simulink model "model_demo"  (R2023b)
settings: Solver=VariableStepAuto  StartTime=0.0  StopTime=10.0  RelTol=1e-3
undefined symbols (not defined in the file): DiscIntNeverNeededParam, magnitude, Newton, Raphson
libraries: simulink x61, slpidlib x19
(part 3 of 3)

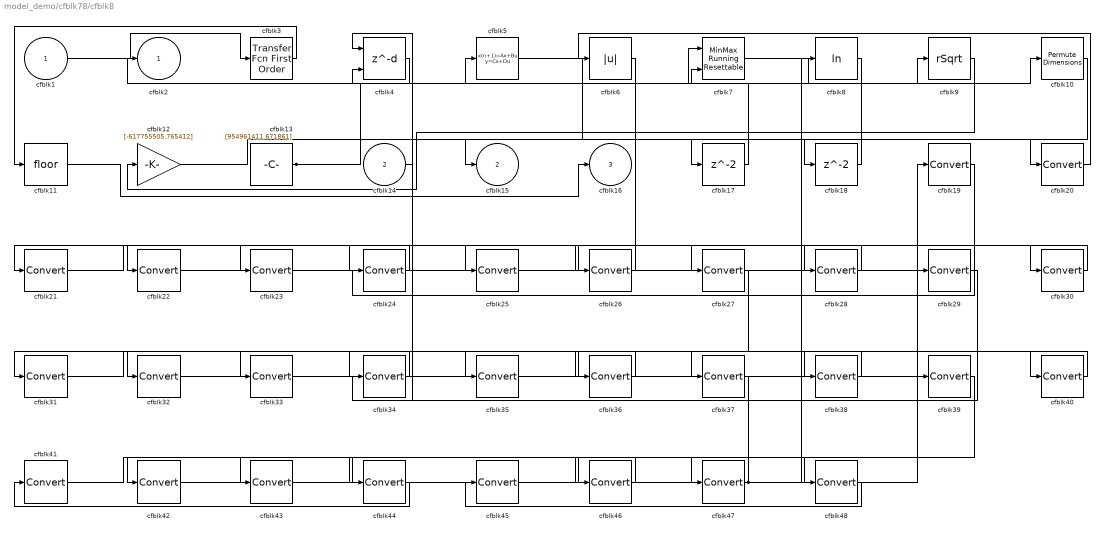
== system model_demo/cfblk78/cfblk8 ==
  cfblk1 : Inport
  cfblk14 : Inport  Port=2
  cfblk10 : PermuteDimensions
  cfblk11 : Rounding
  cfblk12 : Gain  Gain=[-617755505.765412]
  cfblk13 : Constant  Value=[954961411.671861]  SampleTime=1
  cfblk17 : Delay  SampleTime=1
  cfblk18 : Delay  SampleTime=1
  cfblk{19..48} (30 alike) : DataTypeConversion  SaturateOnIntegerOverflow=off  RndMeth=Floor
  cfblk3 : simulink/Discrete/Transfer Fcn First Order  PoleZ=0.95  ICPrevOutput=0.0  DoSatur=off
  cfblk4 : Delay  DelayLengthSource=Input port  SampleTime=1
      settings: InputPortMap=u0,p1
  cfblk5 : DiscreteStateSpace
  cfblk6 : Abs  SaturateOnIntegerOverflow=off
  cfblk7 : simulink/Math Operations/MinMax Running Resettable  Function=min  vinit=0.0
  cfblk8 : Math  Operator=log
  cfblk9 : Sqrt  Operator=rSqrt  AlgorithmType=Newton-Raphson
  cfblk2 : Outport
  cfblk15 : Outport  Port=2
  cfblk16 : Outport  Port=3
  wires:
  cfblk10/1 -> cfblk15/1
  cfblk1/1 -> cfblk3/1
  cfblk4/1 -> cfblk2/1
  cfblk14/1 -> cfblk4/1
  cfblk3/1 -> cfblk11/1
  cfblk7/1 -> cfblk9/1
  cfblk9/1 -> cfblk12/1
  cfblk13/1 -> cfblk10/1, cfblk7/2
  cfblk11/1 -> cfblk16/1
  cfblk8/1 -> cfblk17/1
  cfblk17/1 -> cfblk5/1
  cfblk12/1 -> cfblk18/1
  cfblk18/1 -> cfblk7/1
  cfblk5/1 -> cfblk20/1
  cfblk20/1 -> cfblk6/1
  cfblk6/1 -> cfblk22/1
  cfblk22/1 -> cfblk19/1
  cfblk19/1 -> cfblk24/1
  cfblk24/1 -> cfblk21/1
  cfblk21/1 -> cfblk26/1
  cfblk26/1 -> cfblk23/1
  cfblk23/1 -> cfblk28/1
  cfblk28/1 -> cfblk25/1
  cfblk25/1 -> cfblk30/1
  cfblk30/1 -> cfblk27/1
  cfblk27/1 -> cfblk32/1
  cfblk32/1 -> cfblk29/1
  cfblk29/1 -> cfblk34/1
  cfblk34/1 -> cfblk31/1
  cfblk31/1 -> cfblk36/1
  cfblk36/1 -> cfblk33/1
  cfblk33/1 -> cfblk38/1
  cfblk38/1 -> cfblk35/1
  cfblk35/1 -> cfblk40/1
  cfblk40/1 -> cfblk37/1
  cfblk37/1 -> cfblk42/1
  cfblk42/1 -> cfblk39/1
  cfblk39/1 -> cfblk44/1
  cfblk44/1 -> cfblk41/1
  cfblk45/1 -> cfblk47/1
  cfblk41/1 -> cfblk46/1
  cfblk46/1 -> cfblk43/1
  cfblk47/1 -> cfblk8/1, cfblk4/2
  cfblk43/1 -> cfblk48/1
  cfblk48/1 -> cfblk45/1

== system model_demo/cfblk79/cfblk12 ==
  cfblk1 : Inport
  cfblk3 : simulink/Discrete/Transfer Fcn Real Zero  ZeroZ=0.75  ICPrevInput=0.0  DoSatur=off
  cfblk4 : ComplexToMagnitudeAngle
  cfblk5 : ComplexToMagnitudeAngle
  cfblk6 : Sum  Inputs=--
  cfblk8 : Delay  SampleTime=1
  cfblk2 : Outport
  cfblk7 : Outport  Port=2
  wires:
  cfblk5/1 -> cfblk7/1
  cfblk3/1 -> cfblk4/1
  cfblk5/2 -> cfblk6/1
  cfblk1/1 -> cfblk2/1
  cfblk4/1 -> cfblk5/1
  cfblk4/2 -> cfblk6/2
  cfblk6/1 -> cfblk8/1
  cfblk8/1 -> cfblk3/1

== system model_demo/cfblk80/cfblk6 ==
  cfblk1 : Inport
  cfblk10 : Constant  Value=[956331216.469066]  SampleTime=1
  cfblk12 : Delay  SampleTime=1
  cfblk3 : Delay  DelayLengthSource=Input port  SampleTime=1
      settings: InputPortMap=u0,p1
  cfblk4 : Sum  Inputs=+
  cfblk5 : Sum  Inputs=+
  cfblk6 : Abs  SaturateOnIntegerOverflow=off
  cfblk7 : Sum  Inputs=|++
  cfblk8 : Sqrt
  cfblk9 : Assignment  DiagnosticForDimensions=Warning  IndexOptions=Index vector (dialog)  Indices=1  OutputSizes=1
  cfblk2 : Outport
  cfblk11 : Outport  Port=2
  wires:
  cfblk10/1 -> cfblk8/1, cfblk9/1
  cfblk1/1 -> cfblk3/1
  cfblk5/1 -> cfblk3/2
  cfblk3/1 -> cfblk2/1, cfblk11/1
  cfblk4/1 -> cfblk7/1, cfblk9/2
  cfblk6/1 -> cfblk5/1
  cfblk9/1 -> cfblk7/2
  cfblk8/1 -> cfblk6/1
  cfblk7/1 -> cfblk12/1
  cfblk12/1 -> cfblk4/1

== system model_demo/cfblk80/cfblk7 ==
  cfblk1 : Inport
  cfblk9 : Inport  Port=2
  cfblk10 : Delay  SampleTime=1
  cfblk3 : simulink/Discrete/Transfer Fcn Real Zero  ZeroZ=0.75  ICPrevInput=0.0  DoSatur=off
  cfblk4 : DiscreteZeroPole  Poles=[0 0.5]  Gain=1
  cfblk5 : Delay  SampleTime=1
  cfblk6 : Sum  Inputs=+
  cfblk7 : Sum  Inputs=+
  cfblk8 : Constant  Value=[-3888514.740939]  SampleTime=1
  cfblk2 : Outport
  wires:
  cfblk6/1 -> cfblk2/1
  cfblk1/1 -> cfblk5/1
  cfblk3/1 -> cfblk4/1
  cfblk8/1 -> cfblk6/1
  cfblk4/1 -> cfblk7/1
  cfblk7/1 -> cfblk10/1
  cfblk10/1 -> cfblk3/1

== system model_demo/cfblk80/cfblk8 ==
  cfblk1 : Inport
  cfblk9 : Inport  Port=2
  cfblk10 : Inport  Port=3
  cfblk3 : slpidlib/PID Controller (2DOF)  Controller=PID  Form=Parallel  TimeDomain=Discrete-time  UseExternalTs=off  SampleTime=1  IntegratorMethod=Forward Euler  FilterMethod=Forward Euler  ControllerParametersSource=internal  P=1  I=1  UseKiTs=off  D=0  N=100  UseFilter=on  b=1  c=1  TunerSelectOption=Transfer Function Based (PID Tuner App)  InitialConditionSource=internal  InitialConditionForIntegrator=0  InitialConditionForFilter=0  DifferentiatorICPrevScaledInput=0  ExternalReset=none  TrackingMode=off  Kt=1  LimitOutput=off  SatLimitsSource=internal  UpperSaturationLimit=inf  LowerSaturationLimit=-inf  LinearizeAsGain=off  AntiWindupMode=none  Kb=1  LimitIntegrator=off  UpperIntegratorSaturationLimit=inf  LowerIntegratorSaturationLimit=-inf  POutMin=[]  POutMax=[]  IOutMin=[]  IOutMax=[]  DOutMin=[]  DOutMax=[]  NOutMin=[]  NOutMax=[]  bOutMin=[]  bOutMax=[]  cOutMin=[]  cOutMax=[]  SumOutMin=[]  SumOutMax=[]  SaturationOutMin=[]  SaturationOutMax=[]  PParamMin=[]  PParamMax=[]  IParamMin=[]  IParamMax=[]  DParamMin=[]  DParamMax=[]  NParamMin=[]  NParamMax=[]  bParamMin=[]  bParamMax=[]  cParamMin=[]  cParamMax=[]  KbParamMin=[]  KbParamMax=[]  KtParamMin=[]  KtParamMax=[]  KbOutMin=[]  KbOutMax=[]  KtOutMin=[]  KtOutMax=[]  IntegratorOutMin=[]  IntegratorOutMax=[]  FilterOutMin=[]  FilterOutMax=[]  SumI1OutMin=[]  SumI1OutMax=[]  SumI2OutMin=[]  SumI2OutMax=[]  SumI3OutMin=[]  SumI3OutMax=[]  SumI4OutMin=[]  SumI4OutMax=[]  SumDOutMin=[]  SumDOutMax=[]  Sum1OutMin=[]  Sum1OutMax=[]  Sum2OutMin=[]  Sum2OutMax=[]  Sum3OutMin=[]  Sum3OutMax=[]  DifferentiatorOutMin=[]  DifferentiatorOutMax=[]  FilterDiffOutCoefMin=[]  FilterDiffOutCoefMax=[]  ReciprocalOutMin=[]  ReciprocalOutMax=[]  SumDenOutMin=[]  SumDenOutMax=[]  SumNumOutMin=[]  SumNumOutMax=[]  DivideOutMin=[]  DivideOutMax=[]  UdiffTsProdOutMin=[]  UdiffTsProdOutMax=[]  NTsProdOutMin=[]  NTsProdOutMax=[]  UintegralTsProdOutMin=[]  UintegralTsProdOutMax=[]  UngainTsProdOutMin=[]  UngainTsProdOutMax=[]  ClampingZeroOutDataTypeStr=Inherit: Inherit via back propagation  ClampingZeroOutMin=[]  ClampingZeroOutMax=[]  FilterDenConstantOutDataTypeStr=Inherit: Inherit via back propagation  FilterDenConstantOutMin=[]  FilterDenConstantOutMax=[]  PCopyOutDataTypeStr=Inherit: Inherit via back propagation  PCopyOutMin=[]  PCopyOutMax=[]  NCopyOutDataTypeStr=Inherit: Inherit via back propagation  NCopyOutMin=[]  NCopyOutMax=[]  IntegratorContinuousStateAttributes=''  IntegratorStateMustResolveToSignalObject=off  IntegratorRTWStateStorageClass=Auto  FilterContinuousStateAttributes=''  FilterStateMustResolveToSignalObject=off  FilterRTWStateStorageClass=Auto  ParallelPVariant=InternalParameters  IdealPVariant=Disabled  IVariant=InternalParameters  DVariant=InternalParameters  bVariant=InternalParameters  cVariant=InternalParameters  IntegratorVariant=Discrete  SatVariant=Disabled  AWVariant=Passthrough  PCopyVariant=Disabled  TRVariant=Disabled  FdbkBlocksVariant=Forward  IdealPFdbkVariant=Disabled  SatFdbkVariant=Disabled  DerivativeFilterVariant=ForwardEulerFilter  NVariant=InternalParameters  NCopyVariant=Disabled  FilterICVariant=InternalICsFilter  IntegratorICVariant=InternalICs  ExternalResetVariant=Disabled  TRSumVariant=Passthrough  SumFdbkVariant=Disabled  SumVariant=Sum_PID  TsampFilterVariant=InternalTs  TsampNgainVariant=Passthrough  TsampIntegralVariant=Disabled_SignalSpec  ExternalSaturationOutDataTypeStr=Inherit: Same as second input
      settings: LibrarySourceBlock=simulink/Discrete/Discrete PID Controller (2DOF)
  cfblk4 : Delay  DelayLengthSource=Input port  SampleTime=1
      settings: InputPortMap=u0,p1
  cfblk5 : Sum  Inputs=+
  cfblk6 : MinMax  Function=max  Inputs=3
  cfblk7 : Product  Inputs=*
  cfblk8 : Constant  Value=[999994514.434890]  SampleTime=1
  cfblk2 : Outport
  cfblk11 : Outport  Port=2
  cfblk12 : Outport  Port=3
  wires:
  cfblk6/1 -> cfblk11/1
  cfblk3/1 -> cfblk6/1, cfblk4/2
  cfblk10/1 -> cfblk3/1
  cfblk4/1 -> cfblk12/1
  cfblk7/1 -> cfblk3/2
  cfblk1/1 -> cfblk6/2
  cfblk9/1 -> cfblk4/1, cfblk5/1
  cfblk5/1 -> cfblk6/3, cfblk2/1
  cfblk8/1 -> cfblk7/1

== system model_demo/cfblk80/cfblk9 ==
  cfblk1 : Inport
  cfblk12 : Inport  Port=2
  cfblk13 : Inport  Port=3
  cfblk10 : Constant  Value=[680607672.793325]  SampleTime=1
  cfblk11 : Constant  Value=[263129341.713534]  SampleTime=1
  cfblk3 : PropagationDelay  SampleTime=1
  cfblk4 : UnaryMinus
  cfblk5 : Sqrt
  cfblk6 : Signum
  cfblk7 : PermuteDimensions
  cfblk8 : Trigonometry
  cfblk9 : Constant  Value=[217539892.668750]  SampleTime=1
  cfblk2 : Outport
  wires:
  cfblk7/1 -> cfblk4/1
  cfblk3/1 -> cfblk2/1
  cfblk13/1 -> cfblk5/1
  cfblk4/1 -> cfblk8/1
  cfblk11/1 -> cfblk7/1
  cfblk1/1 -> cfblk3/1
  cfblk12/1 -> cfblk6/1
  cfblk6/1 -> cfblk3/2

== system model_demo/cfblk81/cfblk10 ==
  cfblk1 : Inport
  cfblk6 : Inport  Port=2
  cfblk3 : MinMax  Inputs=3
  cfblk4 : Sum  Inputs=-+
  cfblk5 : Sqrt  Operator=rSqrt  AlgorithmType=Newton-Raphson
  cfblk2 : Outport
  cfblk7 : Outport  Port=2
  wires:
  cfblk4/1 -> cfblk2/1
  cfblk1/1 -> cfblk7/1, cfblk3/3
  cfblk6/1 -> cfblk5/1, cfblk4/2
  cfblk5/1 -> cfblk3/1, cfblk3/2
  cfblk3/1 -> cfblk4/1

== system model_demo/cfblk81/cfblk11 ==
  cfblk1 : Inport
  cfblk8 : Inport  Port=2
  cfblk9 : Inport  Port=3
  cfblk10 : Inport  Port=4
  cfblk3 : simulink/Discrete/Transfer Fcn Lead or Lag  PoleZ=0.95  ZeroZ=0.75  ICPrevOutput=0.0  ICPrevInput=0.0  DoSatur=off
  cfblk4 : Assignment  DiagnosticForDimensions=Warning  IndexOptions=Index vector (dialog)  Indices=1  OutputSizes=1
  cfblk5 : ComplexToRealImag
  cfblk6 : Bias  Bias=[8664871.233920]  SaturateOnIntegerOverflow=off
  cfblk7 : Rounding
  cfblk2 : Outport
  cfblk11 : Outport  Port=2
  wires:
  cfblk6/1 -> cfblk3/1
  cfblk5/1 -> cfblk11/1
  cfblk9/1 -> cfblk2/1
  cfblk10/1 -> cfblk7/1
  cfblk5/2 -> cfblk6/1
  cfblk8/1 -> cfblk4/1
  cfblk1/1 -> cfblk5/1
  cfblk3/1 -> cfblk4/2

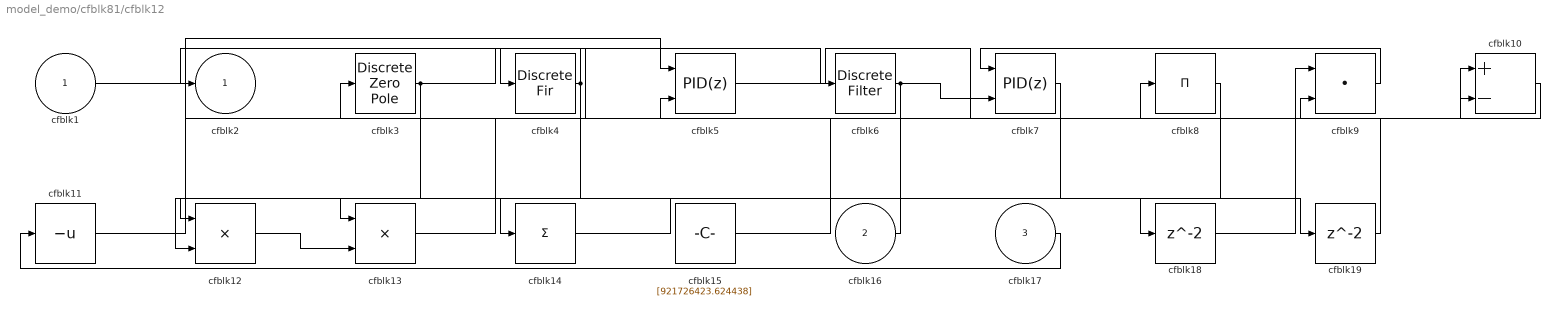
== system model_demo/cfblk81/cfblk12 ==
  cfblk1 : Inport
  cfblk16 : Inport  Port=2
  cfblk17 : Inport  Port=3
  cfblk10 : Sum  Inputs=+-
  cfblk11 : UnaryMinus
  cfblk12 : Product
  cfblk13 : Product
  cfblk14 : Sum  Inputs=+
  cfblk15 : Constant  Value=[921726423.624438]  SampleTime=1
  cfblk18 : Delay  SampleTime=1
  cfblk19 : Delay  SampleTime=1
  cfblk3 : DiscreteZeroPole  Poles=[0 0.5]  Gain=1
  cfblk4 : DiscreteFir  SampleTime=1
  cfblk5 : slpidlib/PID Controller (2DOF)  Controller=PID  Form=Parallel  TimeDomain=Discrete-time  UseExternalTs=off  SampleTime=1  IntegratorMethod=Forward Euler  FilterMethod=Forward Euler  ControllerParametersSource=internal  P=1  I=1  UseKiTs=off  D=0  N=100  UseFilter=on  b=1  c=1  TunerSelectOption=Transfer Function Based (PID Tuner App)  InitialConditionSource=internal  InitialConditionForIntegrator=0  InitialConditionForFilter=0  DifferentiatorICPrevScaledInput=0  ExternalReset=none  TrackingMode=off  Kt=1  LimitOutput=off  SatLimitsSource=internal  UpperSaturationLimit=inf  LowerSaturationLimit=-inf  LinearizeAsGain=off  AntiWindupMode=none  Kb=1  LimitIntegrator=off  UpperIntegratorSaturationLimit=inf  LowerIntegratorSaturationLimit=-inf  POutMin=[]  POutMax=[]  IOutMin=[]  IOutMax=[]  DOutMin=[]  DOutMax=[]  NOutMin=[]  NOutMax=[]  bOutMin=[]  bOutMax=[]  cOutMin=[]  cOutMax=[]  SumOutMin=[]  SumOutMax=[]  SaturationOutMin=[]  SaturationOutMax=[]  PParamMin=[]  PParamMax=[]  IParamMin=[]  IParamMax=[]  DParamMin=[]  DParamMax=[]  NParamMin=[]  NParamMax=[]  bParamMin=[]  bParamMax=[]  cParamMin=[]  cParamMax=[]  KbParamMin=[]  KbParamMax=[]  KtParamMin=[]  KtParamMax=[]  KbOutMin=[]  KbOutMax=[]  KtOutMin=[]  KtOutMax=[]  IntegratorOutMin=[]  IntegratorOutMax=[]  FilterOutMin=[]  FilterOutMax=[]  SumI1OutMin=[]  SumI1OutMax=[]  SumI2OutMin=[]  SumI2OutMax=[]  SumI3OutMin=[]  SumI3OutMax=[]  SumI4OutMin=[]  SumI4OutMax=[]  SumDOutMin=[]  SumDOutMax=[]  Sum1OutMin=[]  Sum1OutMax=[]  Sum2OutMin=[]  Sum2OutMax=[]  Sum3OutMin=[]  Sum3OutMax=[]  DifferentiatorOutMin=[]  DifferentiatorOutMax=[]  FilterDiffOutCoefMin=[]  FilterDiffOutCoefMax=[]  ReciprocalOutMin=[]  ReciprocalOutMax=[]  SumDenOutMin=[]  SumDenOutMax=[]  SumNumOutMin=[]  SumNumOutMax=[]  DivideOutMin=[]  DivideOutMax=[]  UdiffTsProdOutMin=[]  UdiffTsProdOutMax=[]  NTsProdOutMin=[]  NTsProdOutMax=[]  UintegralTsProdOutMin=[]  UintegralTsProdOutMax=[]  UngainTsProdOutMin=[]  UngainTsProdOutMax=[]  ClampingZeroOutDataTypeStr=Inherit: Inherit via back propagation  ClampingZeroOutMin=[]  ClampingZeroOutMax=[]  FilterDenConstantOutDataTypeStr=Inherit: Inherit via back propagation  FilterDenConstantOutMin=[]  FilterDenConstantOutMax=[]  PCopyOutDataTypeStr=Inherit: Inherit via back propagation  PCopyOutMin=[]  PCopyOutMax=[]  NCopyOutDataTypeStr=Inherit: Inherit via back propagation  NCopyOutMin=[]  NCopyOutMax=[]  IntegratorContinuousStateAttributes=''  IntegratorStateMustResolveToSignalObject=off  IntegratorRTWStateStorageClass=Auto  FilterContinuousStateAttributes=''  FilterStateMustResolveToSignalObject=off  FilterRTWStateStorageClass=Auto  ParallelPVariant=InternalParameters  IdealPVariant=Disabled  IVariant=InternalParameters  DVariant=InternalParameters  bVariant=InternalParameters  cVariant=InternalParameters  IntegratorVariant=Discrete  SatVariant=Disabled  AWVariant=Passthrough  PCopyVariant=Disabled  TRVariant=Disabled  FdbkBlocksVariant=Forward  IdealPFdbkVariant=Disabled  SatFdbkVariant=Disabled  DerivativeFilterVariant=ForwardEulerFilter  NVariant=InternalParameters  NCopyVariant=Disabled  FilterICVariant=InternalICsFilter  IntegratorICVariant=InternalICs  ExternalResetVariant=Disabled  TRSumVariant=Passthrough  SumFdbkVariant=Disabled  SumVariant=Sum_PID  TsampFilterVariant=InternalTs  TsampNgainVariant=Passthrough  TsampIntegralVariant=Disabled_SignalSpec  ExternalSaturationOutDataTypeStr=Inherit: Same as second input
      settings: LibrarySourceBlock=simulink/Discrete/Discrete PID Controller (2DOF)
  cfblk6 : DiscreteFilter  SampleTime=1
  cfblk7 : slpidlib/PID Controller (2DOF)  Controller=PID  Form=Parallel  TimeDomain=Discrete-time  UseExternalTs=off  SampleTime=1  IntegratorMethod=Forward Euler  FilterMethod=Forward Euler  ControllerParametersSource=internal  P=1  I=1  UseKiTs=off  D=0  N=100  UseFilter=on  b=1  c=1  TunerSelectOption=Transfer Function Based (PID Tuner App)  InitialConditionSource=internal  InitialConditionForIntegrator=0  InitialConditionForFilter=0  DifferentiatorICPrevScaledInput=0  ExternalReset=none  TrackingMode=off  Kt=1  LimitOutput=off  SatLimitsSource=internal  UpperSaturationLimit=inf  LowerSaturationLimit=-inf  LinearizeAsGain=off  AntiWindupMode=none  Kb=1  LimitIntegrator=off  UpperIntegratorSaturationLimit=inf  LowerIntegratorSaturationLimit=-inf  POutMin=[]  POutMax=[]  IOutMin=[]  IOutMax=[]  DOutMin=[]  DOutMax=[]  NOutMin=[]  NOutMax=[]  bOutMin=[]  bOutMax=[]  cOutMin=[]  cOutMax=[]  SumOutMin=[]  SumOutMax=[]  SaturationOutMin=[]  SaturationOutMax=[]  PParamMin=[]  PParamMax=[]  IParamMin=[]  IParamMax=[]  DParamMin=[]  DParamMax=[]  NParamMin=[]  NParamMax=[]  bParamMin=[]  bParamMax=[]  cParamMin=[]  cParamMax=[]  KbParamMin=[]  KbParamMax=[]  KtParamMin=[]  KtParamMax=[]  KbOutMin=[]  KbOutMax=[]  KtOutMin=[]  KtOutMax=[]  IntegratorOutMin=[]  IntegratorOutMax=[]  FilterOutMin=[]  FilterOutMax=[]  SumI1OutMin=[]  SumI1OutMax=[]  SumI2OutMin=[]  SumI2OutMax=[]  SumI3OutMin=[]  SumI3OutMax=[]  SumI4OutMin=[]  SumI4OutMax=[]  SumDOutMin=[]  SumDOutMax=[]  Sum1OutMin=[]  Sum1OutMax=[]  Sum2OutMin=[]  Sum2OutMax=[]  Sum3OutMin=[]  Sum3OutMax=[]  DifferentiatorOutMin=[]  DifferentiatorOutMax=[]  FilterDiffOutCoefMin=[]  FilterDiffOutCoefMax=[]  ReciprocalOutMin=[]  ReciprocalOutMax=[]  SumDenOutMin=[]  SumDenOutMax=[]  SumNumOutMin=[]  SumNumOutMax=[]  DivideOutMin=[]  DivideOutMax=[]  UdiffTsProdOutMin=[]  UdiffTsProdOutMax=[]  NTsProdOutMin=[]  NTsProdOutMax=[]  UintegralTsProdOutMin=[]  UintegralTsProdOutMax=[]  UngainTsProdOutMin=[]  UngainTsProdOutMax=[]  ClampingZeroOutDataTypeStr=Inherit: Inherit via back propagation  ClampingZeroOutMin=[]  ClampingZeroOutMax=[]  FilterDenConstantOutDataTypeStr=Inherit: Inherit via back propagation  FilterDenConstantOutMin=[]  FilterDenConstantOutMax=[]  PCopyOutDataTypeStr=Inherit: Inherit via back propagation  PCopyOutMin=[]  PCopyOutMax=[]  NCopyOutDataTypeStr=Inherit: Inherit via back propagation  NCopyOutMin=[]  NCopyOutMax=[]  IntegratorContinuousStateAttributes=''  IntegratorStateMustResolveToSignalObject=off  IntegratorRTWStateStorageClass=Auto  FilterContinuousStateAttributes=''  FilterStateMustResolveToSignalObject=off  FilterRTWStateStorageClass=Auto  ParallelPVariant=InternalParameters  IdealPVariant=Disabled  IVariant=InternalParameters  DVariant=InternalParameters  bVariant=InternalParameters  cVariant=InternalParameters  IntegratorVariant=Discrete  SatVariant=Disabled  AWVariant=Passthrough  PCopyVariant=Disabled  TRVariant=Disabled  FdbkBlocksVariant=Forward  IdealPFdbkVariant=Disabled  SatFdbkVariant=Disabled  DerivativeFilterVariant=ForwardEulerFilter  NVariant=InternalParameters  NCopyVariant=Disabled  FilterICVariant=InternalICsFilter  IntegratorICVariant=InternalICs  ExternalResetVariant=Disabled  TRSumVariant=Passthrough  SumFdbkVariant=Disabled  SumVariant=Sum_PID  TsampFilterVariant=InternalTs  TsampNgainVariant=Passthrough  TsampIntegralVariant=Disabled_SignalSpec  ExternalSaturationOutDataTypeStr=Inherit: Same as second input
      settings: LibrarySourceBlock=simulink/Discrete/Discrete PID Controller (2DOF)
  cfblk8 : Product  Inputs=*
  cfblk9 : DotProduct  OutDataTypeStr=Inherit: Inherit via internal rule
  cfblk2 : Outport
  wires:
  cfblk9/1 -> cfblk7/1
  cfblk16/1 -> cfblk4/1
  cfblk5/1 -> cfblk8/1
  cfblk11/1 -> cfblk5/1
  cfblk10/1 -> cfblk5/2
  cfblk3/1 -> cfblk13/1, cfblk6/1
  cfblk1/1 -> cfblk9/2
  cfblk6/1 -> cfblk14/1, cfblk7/2
  cfblk4/1 -> cfblk12/1, cfblk2/1
  cfblk12/1 -> cfblk13/2
  cfblk15/1 -> cfblk10/1
  cfblk13/1 -> cfblk10/2
  cfblk7/1 -> cfblk12/2
  cfblk17/1 -> cfblk11/1
  cfblk8/1 -> cfblk18/1
  cfblk18/1 -> cfblk9/1
  cfblk14/1 -> cfblk19/1
  cfblk19/1 -> cfblk3/1

== system model_demo/cfblk81/cfblk13 ==
  cfblk1 : Inport
  cfblk10 : Inport  Port=2
  cfblk11 : Inport  Port=3
  cfblk14 : Delay  SampleTime=1
  cfblk3 : simulink/Discrete/Transfer Fcn First Order  PoleZ=0.95  ICPrevOutput=0.0  DoSatur=off
  cfblk4 : simulink/Discrete/Transfer Fcn First Order  PoleZ=0.95  ICPrevOutput=0.0  DoSatur=off
  cfblk5 : DiscreteTransferFcn  SampleTime=1
  cfblk6 : simulink/Discrete/Transfer Fcn Real Zero  ZeroZ=0.75  ICPrevInput=0.0  DoSatur=off
  cfblk7 : UnaryMinus
  cfblk8 : Reshape
  cfblk9 : Squeeze
  cfblk2 : Outport
  cfblk12 : Outport  Port=2
  cfblk13 : Outport  Port=3
  wires:
  cfblk4/1 -> cfblk2/1
  cfblk5/1 -> cfblk9/1
  cfblk10/1 -> cfblk12/1
  cfblk6/1 -> cfblk7/1
  cfblk7/1 -> cfblk13/1
  cfblk3/1 -> cfblk6/1
  cfblk11/1 -> cfblk4/1
  cfblk1/1 -> cfblk8/1
  cfblk8/1 -> cfblk3/1
  cfblk9/1 -> cfblk14/1
  cfblk14/1 -> cfblk5/1

== system model_demo/cfblk81/cfblk14 ==
  cfblk1 : Inport
  cfblk14 : Inport  Port=2
  cfblk10 : Polyval  Coefs=[ +2.081618890e-019, -1.441693666e-014, +4.719686976e-010, -8.536869453e-006, +1.621573104e-001, -8.087801117e+001 ]
  cfblk11 : Product  Inputs=**
  cfblk12 : PermuteDimensions
  cfblk13 : Constant  Value=[-781974819.007084]  SampleTime=1
  cfblk3 : slpidlib/PID Controller (2DOF)  Controller=PID  Form=Parallel  TimeDomain=Discrete-time  UseExternalTs=off  SampleTime=1  IntegratorMethod=Forward Euler  FilterMethod=Forward Euler  ControllerParametersSource=internal  P=1  I=1  UseKiTs=off  D=0  N=100  UseFilter=on  b=1  c=1  TunerSelectOption=Transfer Function Based (PID Tuner App)  InitialConditionSource=internal  InitialConditionForIntegrator=0  InitialConditionForFilter=0  DifferentiatorICPrevScaledInput=0  ExternalReset=none  TrackingMode=off  Kt=1  LimitOutput=off  SatLimitsSource=internal  UpperSaturationLimit=inf  LowerSaturationLimit=-inf  LinearizeAsGain=off  AntiWindupMode=none  Kb=1  LimitIntegrator=off  UpperIntegratorSaturationLimit=inf  LowerIntegratorSaturationLimit=-inf  POutMin=[]  POutMax=[]  IOutMin=[]  IOutMax=[]  DOutMin=[]  DOutMax=[]  NOutMin=[]  NOutMax=[]  bOutMin=[]  bOutMax=[]  cOutMin=[]  cOutMax=[]  SumOutMin=[]  SumOutMax=[]  SaturationOutMin=[]  SaturationOutMax=[]  PParamMin=[]  PParamMax=[]  IParamMin=[]  IParamMax=[]  DParamMin=[]  DParamMax=[]  NParamMin=[]  NParamMax=[]  bParamMin=[]  bParamMax=[]  cParamMin=[]  cParamMax=[]  KbParamMin=[]  KbParamMax=[]  KtParamMin=[]  KtParamMax=[]  KbOutMin=[]  KbOutMax=[]  KtOutMin=[]  KtOutMax=[]  IntegratorOutMin=[]  IntegratorOutMax=[]  FilterOutMin=[]  FilterOutMax=[]  SumI1OutMin=[]  SumI1OutMax=[]  SumI2OutMin=[]  SumI2OutMax=[]  SumI3OutMin=[]  SumI3OutMax=[]  SumI4OutMin=[]  SumI4OutMax=[]  SumDOutMin=[]  SumDOutMax=[]  Sum1OutMin=[]  Sum1OutMax=[]  Sum2OutMin=[]  Sum2OutMax=[]  Sum3OutMin=[]  Sum3OutMax=[]  DifferentiatorOutMin=[]  DifferentiatorOutMax=[]  FilterDiffOutCoefMin=[]  FilterDiffOutCoefMax=[]  ReciprocalOutMin=[]  ReciprocalOutMax=[]  SumDenOutMin=[]  SumDenOutMax=[]  SumNumOutMin=[]  SumNumOutMax=[]  DivideOutMin=[]  DivideOutMax=[]  UdiffTsProdOutMin=[]  UdiffTsProdOutMax=[]  NTsProdOutMin=[]  NTsProdOutMax=[]  UintegralTsProdOutMin=[]  UintegralTsProdOutMax=[]  UngainTsProdOutMin=[]  UngainTsProdOutMax=[]  ClampingZeroOutDataTypeStr=Inherit: Inherit via back propagation  ClampingZeroOutMin=[]  ClampingZeroOutMax=[]  FilterDenConstantOutDataTypeStr=Inherit: Inherit via back propagation  FilterDenConstantOutMin=[]  FilterDenConstantOutMax=[]  PCopyOutDataTypeStr=Inherit: Inherit via back propagation  PCopyOutMin=[]  PCopyOutMax=[]  NCopyOutDataTypeStr=Inherit: Inherit via back propagation  NCopyOutMin=[]  NCopyOutMax=[]  IntegratorContinuousStateAttributes=''  IntegratorStateMustResolveToSignalObject=off  IntegratorRTWStateStorageClass=Auto  FilterContinuousStateAttributes=''  FilterStateMustResolveToSignalObject=off  FilterRTWStateStorageClass=Auto  ParallelPVariant=InternalParameters  IdealPVariant=Disabled  IVariant=InternalParameters  DVariant=InternalParameters  bVariant=InternalParameters  cVariant=InternalParameters  IntegratorVariant=Discrete  SatVariant=Disabled  AWVariant=Passthrough  PCopyVariant=Disabled  TRVariant=Disabled  FdbkBlocksVariant=Forward  IdealPFdbkVariant=Disabled  SatFdbkVariant=Disabled  DerivativeFilterVariant=ForwardEulerFilter  NVariant=InternalParameters  NCopyVariant=Disabled  FilterICVariant=InternalICsFilter  IntegratorICVariant=InternalICs  ExternalResetVariant=Disabled  TRSumVariant=Passthrough  SumFdbkVariant=Disabled  SumVariant=Sum_PID  TsampFilterVariant=InternalTs  TsampNgainVariant=Passthrough  TsampIntegralVariant=Disabled_SignalSpec  ExternalSaturationOutDataTypeStr=Inherit: Same as second input
      settings: LibrarySourceBlock=simulink/Discrete/Discrete PID Controller (2DOF)
  cfblk4 : simulink/Discrete/Transfer Fcn Real Zero  ZeroZ=0.75  ICPrevInput=0.0  DoSatur=off
  cfblk5 : DiscreteZeroPole  Poles=[0 0.5]  Gain=1
  cfblk6 : DiscreteStateSpace
  cfblk7 : Abs  SaturateOnIntegerOverflow=off
  cfblk8 : Trigonometry
  cfblk9 : Math  Operator=log10
  cfblk2 : Outport
  cfblk15 : Outport  Port=2
  cfblk16 : Outport  Port=3
  wires:
  cfblk13/1 -> cfblk11/1, cfblk12/1
  cfblk8/1 -> cfblk4/1
  cfblk3/1 -> cfblk6/1
  cfblk12/1 -> cfblk10/1
  cfblk7/1 -> cfblk2/1
  cfblk5/1 -> cfblk16/1, cfblk3/2
  cfblk6/1 -> cfblk15/1
  cfblk9/1 -> cfblk7/1
  cfblk1/1 -> cfblk11/2
  cfblk14/1 -> cfblk5/1
  cfblk10/1 -> cfblk9/1
  cfblk11/1 -> cfblk8/1
  cfblk4/1 -> cfblk3/1

== system model_demo/cfblk81/cfblk9 ==
  cfblk1 : Inport
  cfblk7 : Inport  Port=2
  cfblk8 : Inport  Port=3
  cfblk10 : Delay  SampleTime=1
  cfblk3 : simulink/Discrete/Transfer Fcn Lead or Lag  PoleZ=0.95  ZeroZ=0.75  ICPrevOutput=0.0  ICPrevInput=0.0  DoSatur=off
  cfblk4 : Sin  TimeSource=Use external signal  SampleTime=0
  cfblk5 : Abs  SaturateOnIntegerOverflow=off
  cfblk6 : MinMax  Function=max  Inputs=3
  cfblk2 : Outport
  cfblk9 : Outport  Port=2
  wires:
  cfblk7/1 -> cfblk2/1
  cfblk3/1 -> cfblk4/1
  cfblk5/1 -> cfblk9/1, cfblk10/1
  cfblk8/1 -> cfblk6/1
  cfblk6/1 -> cfblk5/1
  cfblk4/1 -> cfblk6/2
  cfblk1/1 -> cfblk3/1
  cfblk10/1 -> cfblk6/3

== system model_demo/cfblk82/cfblk12 ==
  cfblk1 : Inport
  cfblk11 : Inport  Port=2
  cfblk12 : Inport  Port=3
  cfblk13 : Inport  Port=4
  cfblk14 : Inport  Port=5
  cfblk15 : Inport  Port=6
  cfblk10 : Constant  Value=[345707446.991535]  SampleTime=1
  cfblk3 : Delay  ShowEnablePort=on  SampleTime=1
      settings: InputPortMap=u0,e6
  cfblk4 : simulink/Discrete/Transfer Fcn First Order  PoleZ=0.95  ICPrevOutput=0.0  DoSatur=off
  cfblk5 : slpidlib/PID Controller (2DOF)  Controller=PID  Form=Parallel  TimeDomain=Discrete-time  UseExternalTs=off  SampleTime=1  IntegratorMethod=Forward Euler  FilterMethod=Forward Euler  ControllerParametersSource=internal  P=1  I=1  UseKiTs=off  D=0  N=100  UseFilter=on  b=1  c=1  TunerSelectOption=Transfer Function Based (PID Tuner App)  InitialConditionSource=internal  InitialConditionForIntegrator=0  InitialConditionForFilter=0  DifferentiatorICPrevScaledInput=0  ExternalReset=none  TrackingMode=off  Kt=1  LimitOutput=off  SatLimitsSource=internal  UpperSaturationLimit=inf  LowerSaturationLimit=-inf  LinearizeAsGain=off  AntiWindupMode=none  Kb=1  LimitIntegrator=off  UpperIntegratorSaturationLimit=inf  LowerIntegratorSaturationLimit=-inf  POutMin=[]  POutMax=[]  IOutMin=[]  IOutMax=[]  DOutMin=[]  DOutMax=[]  NOutMin=[]  NOutMax=[]  bOutMin=[]  bOutMax=[]  cOutMin=[]  cOutMax=[]  SumOutMin=[]  SumOutMax=[]  SaturationOutMin=[]  SaturationOutMax=[]  PParamMin=[]  PParamMax=[]  IParamMin=[]  IParamMax=[]  DParamMin=[]  DParamMax=[]  NParamMin=[]  NParamMax=[]  bParamMin=[]  bParamMax=[]  cParamMin=[]  cParamMax=[]  KbParamMin=[]  KbParamMax=[]  KtParamMin=[]  KtParamMax=[]  KbOutMin=[]  KbOutMax=[]  KtOutMin=[]  KtOutMax=[]  IntegratorOutMin=[]  IntegratorOutMax=[]  FilterOutMin=[]  FilterOutMax=[]  SumI1OutMin=[]  SumI1OutMax=[]  SumI2OutMin=[]  SumI2OutMax=[]  SumI3OutMin=[]  SumI3OutMax=[]  SumI4OutMin=[]  SumI4OutMax=[]  SumDOutMin=[]  SumDOutMax=[]  Sum1OutMin=[]  Sum1OutMax=[]  Sum2OutMin=[]  Sum2OutMax=[]  Sum3OutMin=[]  Sum3OutMax=[]  DifferentiatorOutMin=[]  DifferentiatorOutMax=[]  FilterDiffOutCoefMin=[]  FilterDiffOutCoefMax=[]  ReciprocalOutMin=[]  ReciprocalOutMax=[]  SumDenOutMin=[]  SumDenOutMax=[]  SumNumOutMin=[]  SumNumOutMax=[]  DivideOutMin=[]  DivideOutMax=[]  UdiffTsProdOutMin=[]  UdiffTsProdOutMax=[]  NTsProdOutMin=[]  NTsProdOutMax=[]  UintegralTsProdOutMin=[]  UintegralTsProdOutMax=[]  UngainTsProdOutMin=[]  UngainTsProdOutMax=[]  ClampingZeroOutDataTypeStr=Inherit: Inherit via back propagation  ClampingZeroOutMin=[]  ClampingZeroOutMax=[]  FilterDenConstantOutDataTypeStr=Inherit: Inherit via back propagation  FilterDenConstantOutMin=[]  FilterDenConstantOutMax=[]  PCopyOutDataTypeStr=Inherit: Inherit via back propagation  PCopyOutMin=[]  PCopyOutMax=[]  NCopyOutDataTypeStr=Inherit: Inherit via back propagation  NCopyOutMin=[]  NCopyOutMax=[]  IntegratorContinuousStateAttributes=''  IntegratorStateMustResolveToSignalObject=off  IntegratorRTWStateStorageClass=Auto  FilterContinuousStateAttributes=''  FilterStateMustResolveToSignalObject=off  FilterRTWStateStorageClass=Auto  ParallelPVariant=InternalParameters  IdealPVariant=Disabled  IVariant=InternalParameters  DVariant=InternalParameters  bVariant=InternalParameters  cVariant=InternalParameters  IntegratorVariant=Discrete  SatVariant=Disabled  AWVariant=Passthrough  PCopyVariant=Disabled  TRVariant=Disabled  FdbkBlocksVariant=Forward  IdealPFdbkVariant=Disabled  SatFdbkVariant=Disabled  DerivativeFilterVariant=ForwardEulerFilter  NVariant=InternalParameters  NCopyVariant=Disabled  FilterICVariant=InternalICsFilter  IntegratorICVariant=InternalICs  ExternalResetVariant=Disabled  TRSumVariant=Passthrough  SumFdbkVariant=Disabled  SumVariant=Sum_PID  TsampFilterVariant=InternalTs  TsampNgainVariant=Passthrough  TsampIntegralVariant=Disabled_SignalSpec  ExternalSaturationOutDataTypeStr=Inherit: Same as second input
      settings: LibrarySourceBlock=simulink/Discrete/Discrete PID Controller (2DOF)
  cfblk6 : Sum  Inputs=+-
  cfblk7 : Product  Inputs=**
  cfblk8 : Product
  cfblk9 : Constant  Value=[806755621.526693]  SampleTime=1
  cfblk2 : Outport
  cfblk16 : Outport  Port=2
  wires:
  cfblk9/1 -> cfblk8/1
  cfblk14/1 -> cfblk6/1
  cfblk1/1 -> cfblk4/1
  cfblk4/1 -> cfblk16/1
  cfblk5/1 -> cfblk2/1
  cfblk7/1 -> cfblk6/2
  cfblk12/1 -> cfblk8/2
  cfblk11/1 -> cfblk7/1
  cfblk6/1 -> cfblk3/1
  cfblk13/1 -> cfblk7/2
  cfblk3/1 -> cfblk5/1
  cfblk15/1 -> cfblk5/2
  cfblk8/1 -> cfblk3/2

== system model_demo/cfblk82/cfblk13 ==
  cfblk1 : Inport
  cfblk6 : Inport  Port=2
  cfblk3 : simulink/Discrete/Transfer Fcn First Order  PoleZ=0.95  ICPrevOutput=0.0  DoSatur=off
  cfblk4 : simulink/Discrete/Transfer Fcn Lead or Lag  PoleZ=0.95  ZeroZ=0.75  ICPrevOutput=0.0  ICPrevInput=0.0  DoSatur=off
  cfblk5 : simulink/Math Operations/Slider Gain  gain=1  low=0  high=2
  cfblk2 : Outport
  cfblk7 : Outport  Port=2
  wires:
  cfblk4/1 -> cfblk5/1
  cfblk5/1 -> cfblk2/1
  cfblk6/1 -> cfblk3/1
  cfblk1/1 -> cfblk7/1
  cfblk3/1 -> cfblk4/1

== system model_demo/cfblk82/cfblk14 ==
  cfblk1 : Inport
  cfblk7 : Inport  Port=2
  cfblk8 : Inport  Port=3
  cfblk9 : Inport  Port=4
  cfblk10 : Delay  SampleTime=1
  cfblk3 : Delay  DelayLengthSource=Input port  SampleTime=1
      settings: InputPortMap=u0,p1
  cfblk4 : Delay  DelayLengthSource=Input port  SampleTime=1
      settings: InputPortMap=u0,p1
  cfblk5 : Polyval  Coefs=[ +2.081618890e-019, -1.441693666e-014, +4.719686976e-010, -8.536869453e-006, +1.621573104e-001, -8.087801117e+001 ]
  cfblk6 : Gain  Gain=[424032298.343210]
  cfblk2 : Outport
  wires:
  cfblk8/1 -> cfblk2/1
  cfblk5/1 -> cfblk4/1
  cfblk1/1 -> cfblk4/2
  cfblk7/1 -> cfblk5/1
  cfblk3/1 -> cfblk6/1
  cfblk9/1 -> cfblk3/2
  cfblk6/1 -> cfblk10/1
  cfblk10/1 -> cfblk3/1

== system model_demo/cfblk82/cfblk18 ==
  cfblk1 : Inport
  cfblk7 : Inport  Port=2
  cfblk8 : Inport  Port=3
  Action Port : ActionPort  ActionPortLabel=if(u1 >= 0)
  cfblk3 : simulink/Discrete/Difference  ICPrevInput=0.0  OutMin=[]  OutMax=[]  OutDataTypeStr=Inherit: Inherit via back propagation  OutDataType=fixdt(1, 16)  OutScaling=2^-10  DoSatur=off
  cfblk4 : slpidlib/PID Controller (2DOF)  Controller=PID  Form=Parallel  TimeDomain=Discrete-time  UseExternalTs=off  SampleTime=-1  IntegratorMethod=Forward Euler  FilterMethod=Forward Euler  ControllerParametersSource=internal  P=1  I=1  UseKiTs=off  D=0  N=100  UseFilter=on  b=1  c=1  TunerSelectOption=Transfer Function Based (PID Tuner App)  InitialConditionSource=internal  InitialConditionForIntegrator=0  InitialConditionForFilter=0  DifferentiatorICPrevScaledInput=0  ExternalReset=none  TrackingMode=off  Kt=1  LimitOutput=off  SatLimitsSource=internal  UpperSaturationLimit=inf  LowerSaturationLimit=-inf  LinearizeAsGain=off  AntiWindupMode=none  Kb=1  LimitIntegrator=off  UpperIntegratorSaturationLimit=inf  LowerIntegratorSaturationLimit=-inf  POutMin=[]  POutMax=[]  IOutMin=[]  IOutMax=[]  DOutMin=[]  DOutMax=[]  NOutMin=[]  NOutMax=[]  bOutMin=[]  bOutMax=[]  cOutMin=[]  cOutMax=[]  SumOutMin=[]  SumOutMax=[]  SaturationOutMin=[]  SaturationOutMax=[]  PParamMin=[]  PParamMax=[]  IParamMin=[]  IParamMax=[]  DParamMin=[]  DParamMax=[]  NParamMin=[]  NParamMax=[]  bParamMin=[]  bParamMax=[]  cParamMin=[]  cParamMax=[]  KbParamMin=[]  KbParamMax=[]  KtParamMin=[]  KtParamMax=[]  KbOutMin=[]  KbOutMax=[]  KtOutMin=[]  KtOutMax=[]  IntegratorOutMin=[]  IntegratorOutMax=[]  FilterOutMin=[]  FilterOutMax=[]  SumI1OutMin=[]  SumI1OutMax=[]  SumI2OutMin=[]  SumI2OutMax=[]  SumI3OutMin=[]  SumI3OutMax=[]  SumI4OutMin=[]  SumI4OutMax=[]  SumDOutMin=[]  SumDOutMax=[]  Sum1OutMin=[]  Sum1OutMax=[]  Sum2OutMin=[]  Sum2OutMax=[]  Sum3OutMin=[]  Sum3OutMax=[]  DifferentiatorOutMin=[]  DifferentiatorOutMax=[]  FilterDiffOutCoefMin=[]  FilterDiffOutCoefMax=[]  ReciprocalOutMin=[]  ReciprocalOutMax=[]  SumDenOutMin=[]  SumDenOutMax=[]  SumNumOutMin=[]  SumNumOutMax=[]  DivideOutMin=[]  DivideOutMax=[]  UdiffTsProdOutMin=[]  UdiffTsProdOutMax=[]  NTsProdOutMin=[]  NTsProdOutMax=[]  UintegralTsProdOutMin=[]  UintegralTsProdOutMax=[]  UngainTsProdOutMin=[]  UngainTsProdOutMax=[]  ClampingZeroOutDataTypeStr=Inherit: Inherit via back propagation  ClampingZeroOutMin=[]  ClampingZeroOutMax=[]  FilterDenConstantOutDataTypeStr=Inherit: Inherit via back propagation  FilterDenConstantOutMin=[]  FilterDenConstantOutMax=[]  PCopyOutDataTypeStr=Inherit: Inherit via back propagation  PCopyOutMin=[]  PCopyOutMax=[]  NCopyOutDataTypeStr=Inherit: Inherit via back propagation  NCopyOutMin=[]  NCopyOutMax=[]  IntegratorContinuousStateAttributes=''  IntegratorStateMustResolveToSignalObject=off  IntegratorRTWStateStorageClass=Auto  FilterContinuousStateAttributes=''  FilterStateMustResolveToSignalObject=off  FilterRTWStateStorageClass=Auto  ParallelPVariant=InternalParameters  IdealPVariant=Disabled  IVariant=InternalParameters  DVariant=InternalParameters  bVariant=InternalParameters  cVariant=InternalParameters  IntegratorVariant=Discrete  SatVariant=Disabled  AWVariant=Passthrough  PCopyVariant=Disabled  TRVariant=Disabled  FdbkBlocksVariant=Forward  IdealPFdbkVariant=Disabled  SatFdbkVariant=Disabled  DerivativeFilterVariant=ForwardEulerFilter  NVariant=InternalParameters  NCopyVariant=Disabled  FilterICVariant=InternalICsFilter  IntegratorICVariant=InternalICs  ExternalResetVariant=Disabled  TRSumVariant=Passthrough  SumFdbkVariant=Disabled  SumVariant=Sum_PID  TsampFilterVariant=InternalTs  TsampNgainVariant=Passthrough  TsampIntegralVariant=Disabled_SignalSpec  ExternalSaturationOutDataTypeStr=Inherit: Same as second input
      settings: LibrarySourceBlock=simulink/Discrete/Discrete PID Controller (2DOF)
  cfblk5 : Squeeze
  cfblk6 : Sum  Inputs=--
  cfblk2 : Outport
  wires:
  cfblk3/1 -> cfblk4/1
  cfblk1/1 -> cfblk2/1
  cfblk8/1 -> cfblk6/1
  cfblk5/1 -> cfblk6/2
  cfblk7/1 -> cfblk5/1, cfblk4/2
  cfblk6/1 -> cfblk3/1

== system model_demo/cfblk82/cfblk19 ==
  cfblk1 : Inport
  cfblk5 : Inport  Port=2
  cfblk6 : Inport  Port=3
  Action Port : ActionPort  ActionPortLabel=else
  cfblk3 : Delay
  cfblk4 : slpidlib/PID Controller  Controller=PID  Form=Parallel  TimeDomain=Discrete-time  UseExternalTs=off  SampleTime=-1  IntegratorMethod=Forward Euler  FilterMethod=Forward Euler  ControllerParametersSource=internal  P=1  I=1  UseKiTs=off  D=0  N=100  UseFilter=on  TunerSelectOption=Transfer Function Based (PID Tuner App)  InitialConditionSource=internal  InitialConditionForIntegrator=0  InitialConditionForFilter=0  DifferentiatorICPrevScaledInput=0  ExternalReset=none  TrackingMode=off  Kt=1  LimitOutput=off  SatLimitsSource=internal  UpperSaturationLimit=inf  LowerSaturationLimit=-inf  LinearizeAsGain=off  AntiWindupMode=none  Kb=1  LimitIntegrator=off  UpperIntegratorSaturationLimit=inf  LowerIntegratorSaturationLimit=-inf  POutMin=[]  POutMax=[]  IOutMin=[]  IOutMax=[]  DOutMin=[]  DOutMax=[]  NOutMin=[]  NOutMax=[]  SumOutMin=[]  SumOutMax=[]  SaturationOutMin=[]  SaturationOutMax=[]  PParamMin=[]  PParamMax=[]  IParamMin=[]  IParamMax=[]  DParamMin=[]  DParamMax=[]  NParamMin=[]  NParamMax=[]  KbParamMin=[]  KbParamMax=[]  KtParamMin=[]  KtParamMax=[]  KbOutMin=[]  KbOutMax=[]  KtOutMin=[]  KtOutMax=[]  IntegratorOutMin=[]  IntegratorOutMax=[]  FilterOutMin=[]  FilterOutMax=[]  SumI1OutMin=[]  SumI1OutMax=[]  SumI2OutMin=[]  SumI2OutMax=[]  SumI3OutMin=[]  SumI3OutMax=[]  SumI4OutMin=[]  SumI4OutMax=[]  SumDOutMin=[]  SumDOutMax=[]  DifferentiatorOutMin=[]  DifferentiatorOutMax=[]  FilterDiffOutCoefMin=[]  FilterDiffOutCoefMax=[]  ReciprocalOutMin=[]  ReciprocalOutMax=[]  SumDenOutMin=[]  SumDenOutMax=[]  SumNumOutMin=[]  SumNumOutMax=[]  DivideOutMin=[]  DivideOutMax=[]  UdiffTsProdOutMin=[]  UdiffTsProdOutMax=[]  NTsProdOutMin=[]  NTsProdOutMax=[]  UintegralTsProdOutMin=[]  UintegralTsProdOutMax=[]  UngainTsProdOutMin=[]  UngainTsProdOutMax=[]  ClampingZeroOutDataTypeStr=Inherit: Inherit via back propagation  ClampingZeroOutMin=[]  ClampingZeroOutMax=[]  FilterDenConstantOutDataTypeStr=Inherit: Inherit via back propagation  FilterDenConstantOutMin=[]  FilterDenConstantOutMax=[]  PCopyOutDataTypeStr=Inherit: Inherit via back propagation  PCopyOutMin=[]  PCopyOutMax=[]  NCopyOutDataTypeStr=Inherit: Inherit via back propagation  NCopyOutMin=[]  NCopyOutMax=[]  IntegratorContinuousStateAttributes=''  IntegratorStateMustResolveToSignalObject=off  IntegratorRTWStateStorageClass=Auto  FilterContinuousStateAttributes=''  FilterStateMustResolveToSignalObject=off  FilterRTWStateStorageClass=Auto  ParallelPVariant=InternalParameters  IdealPVariant=Disabled  IVariant=InternalParameters  DVariant=InternalParameters  IntegratorVariant=Discrete  SatVariant=Disabled  AWVariant=Passthrough  PCopyVariant=Disabled  TRVariant=Disabled  FdbkBlocksVariant=Forward  IdealPFdbkVariant=Disabled  SatFdbkVariant=Disabled  DerivativeFilterVariant=ForwardEulerFilter  NVariant=InternalParameters  NCopyVariant=Disabled  FilterICVariant=InternalICsFilter  IntegratorICVariant=InternalICs  ExternalResetVariant=Disabled  TRSumVariant=Passthrough  SumFdbkVariant=Disabled  SumVariant=Sum_PID  TsampFilterVariant=InternalTs  TsampNgainVariant=Passthrough  TsampIntegralVariant=Disabled_SignalSpec  ExternalSaturationOutDataTypeStr=Inherit: Same as second input
      settings: LibrarySourceBlock=simulink/Discrete/Discrete PID Controller
  cfblk2 : Outport
  cfblk7 : Outport  Port=2
  wires:
  cfblk6/1 -> cfblk3/1
  cfblk5/1 -> cfblk7/1
  cfblk4/1 -> cfblk2/1
  cfblk3/1 -> cfblk4/1

== system model_demo/cfblk83/cfblk7 ==
  cfblk1 : Inport
  cfblk9 : Inport  Port=2
  cfblk10 : Inport  Port=3
  cfblk11 : Inport  Port=4
  cfblk12 : Inport  Port=5
  cfblk3 : simulink/Discrete/Transfer Fcn Lead or Lag  PoleZ=0.95  ZeroZ=0.75  ICPrevOutput=0.0  ICPrevInput=0.0  DoSatur=off
  cfblk4 : simulink/Discrete/Difference  ICPrevInput=0.0  OutMin=[]  OutMax=[]  OutDataTypeStr=Inherit: Inherit via back propagation  OutDataType=fixdt(1, 16)  OutScaling=2^-10  DoSatur=off
  cfblk5 : DotProduct  OutDataTypeStr=Inherit: Inherit via internal rule
  cfblk6 : Signum
  cfblk7 : Constant  Value=[-754686844.111725]  SampleTime=1
  cfblk8 : Constant  Value=[225282182.475113]  SampleTime=1
  cfblk2 : Outport
  wires:
  cfblk10/1 -> cfblk6/1
  cfblk5/1 -> cfblk4/1
  cfblk1/1 -> cfblk5/1
  cfblk8/1 -> cfblk2/1
  cfblk4/1 -> cfblk3/1
  cfblk12/1 -> cfblk5/2

== system model_demo/cfblk83/cfblk8 ==
  cfblk1 : Inport
  cfblk8 : Inport  Port=2
  cfblk3 : Delay  DelayLengthSource=Input port  SampleTime=1
      settings: InputPortMap=u0,p1
  cfblk4 : DiscreteStateSpace
  cfblk5 : PropagationDelay  SampleTime=1
  cfblk6 : Abs  SaturateOnIntegerOverflow=off
  cfblk7 : Reshape
  cfblk9 : Delay  SampleTime=1
  cfblk2 : Outport
  wires:
  cfblk1/1 -> cfblk2/1
  cfblk4/1 -> cfblk7/1
  cfblk8/1 -> cfblk4/1
  cfblk3/1 -> cfblk5/1
  cfblk5/1 -> cfblk6/1
  cfblk7/1 -> cfblk3/1, cfblk3/2
  cfblk6/1 -> cfblk9/1
  cfblk9/1 -> cfblk5/2

== system model_demo/cfblk85/cfblk6 ==
  cfblk1 : Inport
  cfblk10 : Inport  Port=2
  cfblk11 : Inport  Port=3
  cfblk12 : Inport  Port=4
  cfblk14 : Delay
  cfblk3 : UnitDelay  SampleTime=-1  HasFrameUpgradeWarning=on
  cfblk4 : Polyval  Coefs=[ +2.081618890e-019, -1.441693666e-014, +4.719686976e-010, -8.536869453e-006, +1.621573104e-001, -8.087801117e+001 ]
  cfblk5 : Sqrt
  cfblk6 : PermuteDimensions
  cfblk7 : Sum  Inputs=+-
  cfblk8 : Sum  Inputs=|++
  cfblk9 : Constant  Value=[970697430.648301]  SampleTime=1
  cfblk2 : Outport
  cfblk13 : Outport  Port=2
  wires:
  cfblk9/1 -> cfblk13/1
  cfblk8/1 -> cfblk7/1
  cfblk4/1 -> cfblk6/1
  cfblk10/1 -> cfblk2/1
  cfblk12/1 -> cfblk7/2
  cfblk7/1 -> cfblk4/1
  cfblk11/1 -> cfblk8/1
  cfblk5/1 -> cfblk8/2
  cfblk3/1 -> cfblk5/1
  cfblk6/1 -> cfblk14/1
  cfblk14/1 -> cfblk3/1

== system model_demo/cfblk85/cfblk7 ==
  cfblk1 : Inport
  cfblk5 : Inport  Port=2
  cfblk6 : Inport  Port=3
  cfblk3 : UnaryMinus
  cfblk4 : Sum  Inputs=+-
  cfblk2 : Outport
  cfblk7 : Outport  Port=2
  wires:
  cfblk5/1 -> cfblk3/1
  cfblk6/1 -> cfblk4/1
  cfblk1/1 -> cfblk4/2
  cfblk4/1 -> cfblk2/1
  cfblk3/1 -> cfblk7/1

== system model_demo/cfblk85/cfblk8 ==
  cfblk1 : Inport
  cfblk10 : Inport  Port=2
  cfblk13 : Delay
  cfblk14 : Delay
  cfblk3 : DiscreteIntegrator  SampleTime=-1  ICPrevOutput=DiscIntNeverNeededParam  ICPrevScaledInput=DiscIntNeverNeededParam
  cfblk4 : Delay  DelayLengthSource=Input port
      settings: InputPortMap=u0,p1
  cfblk5 : DiscreteIntegrator  SampleTime=-1  ICPrevOutput=DiscIntNeverNeededParam  ICPrevScaledInput=DiscIntNeverNeededParam
  cfblk6 : Product
  cfblk7 : Signum
  cfblk8 : Rounding
  cfblk9 : Constant  Value=[715463942.614666]  SampleTime=1
  cfblk2 : Outport
  cfblk11 : Outport  Port=2
  cfblk12 : Outport  Port=3
  wires:
  cfblk3/1 -> cfblk7/1
  cfblk10/1 -> cfblk11/1
  cfblk7/1 -> cfblk8/1
  cfblk1/1 -> cfblk4/2
  cfblk4/1 -> cfblk3/1
  cfblk5/1 -> cfblk12/1, cfblk6/2
  cfblk9/1 -> cfblk2/1, cfblk6/1
  cfblk8/1 -> cfblk13/1
  cfblk13/1 -> cfblk4/1
  cfblk6/1 -> cfblk14/1
  cfblk14/1 -> cfblk5/1

== system model_demo/cfblk86/cfblk6 ==
  cfblk1 : Inport
  cfblk8 : Inport  Port=2
  cfblk9 : Inport  Port=3
  cfblk10 : Inport  Port=4
  cfblk11 : Inport  Port=5
  cfblk12 : Inport  Port=6
  cfblk3 : slpidlib/PID Controller  Controller=PID  Form=Parallel  TimeDomain=Discrete-time  UseExternalTs=off  SampleTime=-1  IntegratorMethod=Forward Euler  FilterMethod=Forward Euler  ControllerParametersSource=internal  P=1  I=1  UseKiTs=off  D=0  N=100  UseFilter=on  TunerSelectOption=Transfer Function Based (PID Tuner App)  InitialConditionSource=internal  InitialConditionForIntegrator=0  InitialConditionForFilter=0  DifferentiatorICPrevScaledInput=0  ExternalReset=none  TrackingMode=off  Kt=1  LimitOutput=off  SatLimitsSource=internal  UpperSaturationLimit=inf  LowerSaturationLimit=-inf  LinearizeAsGain=off  AntiWindupMode=none  Kb=1  LimitIntegrator=off  UpperIntegratorSaturationLimit=inf  LowerIntegratorSaturationLimit=-inf  POutMin=[]  POutMax=[]  IOutMin=[]  IOutMax=[]  DOutMin=[]  DOutMax=[]  NOutMin=[]  NOutMax=[]  SumOutMin=[]  SumOutMax=[]  SaturationOutMin=[]  SaturationOutMax=[]  PParamMin=[]  PParamMax=[]  IParamMin=[]  IParamMax=[]  DParamMin=[]  DParamMax=[]  NParamMin=[]  NParamMax=[]  KbParamMin=[]  KbParamMax=[]  KtParamMin=[]  KtParamMax=[]  KbOutMin=[]  KbOutMax=[]  KtOutMin=[]  KtOutMax=[]  IntegratorOutMin=[]  IntegratorOutMax=[]  FilterOutMin=[]  FilterOutMax=[]  SumI1OutMin=[]  SumI1OutMax=[]  SumI2OutMin=[]  SumI2OutMax=[]  SumI3OutMin=[]  SumI3OutMax=[]  SumI4OutMin=[]  SumI4OutMax=[]  SumDOutMin=[]  SumDOutMax=[]  DifferentiatorOutMin=[]  DifferentiatorOutMax=[]  FilterDiffOutCoefMin=[]  FilterDiffOutCoefMax=[]  ReciprocalOutMin=[]  ReciprocalOutMax=[]  SumDenOutMin=[]  SumDenOutMax=[]  SumNumOutMin=[]  SumNumOutMax=[]  DivideOutMin=[]  DivideOutMax=[]  UdiffTsProdOutMin=[]  UdiffTsProdOutMax=[]  NTsProdOutMin=[]  NTsProdOutMax=[]  UintegralTsProdOutMin=[]  UintegralTsProdOutMax=[]  UngainTsProdOutMin=[]  UngainTsProdOutMax=[]  ClampingZeroOutDataTypeStr=Inherit: Inherit via back propagation  ClampingZeroOutMin=[]  ClampingZeroOutMax=[]  FilterDenConstantOutDataTypeStr=Inherit: Inherit via back propagation  FilterDenConstantOutMin=[]  FilterDenConstantOutMax=[]  PCopyOutDataTypeStr=Inherit: Inherit via back propagation  PCopyOutMin=[]  PCopyOutMax=[]  NCopyOutDataTypeStr=Inherit: Inherit via back propagation  NCopyOutMin=[]  NCopyOutMax=[]  IntegratorContinuousStateAttributes=''  IntegratorStateMustResolveToSignalObject=off  IntegratorRTWStateStorageClass=Auto  FilterContinuousStateAttributes=''  FilterStateMustResolveToSignalObject=off  FilterRTWStateStorageClass=Auto  ParallelPVariant=InternalParameters  IdealPVariant=Disabled  IVariant=InternalParameters  DVariant=InternalParameters  IntegratorVariant=Discrete  SatVariant=Disabled  AWVariant=Passthrough  PCopyVariant=Disabled  TRVariant=Disabled  FdbkBlocksVariant=Forward  IdealPFdbkVariant=Disabled  SatFdbkVariant=Disabled  DerivativeFilterVariant=ForwardEulerFilter  NVariant=InternalParameters  NCopyVariant=Disabled  FilterICVariant=InternalICsFilter  IntegratorICVariant=InternalICs  ExternalResetVariant=Disabled  TRSumVariant=Passthrough  SumFdbkVariant=Disabled  SumVariant=Sum_PID  TsampFilterVariant=InternalTs  TsampNgainVariant=Passthrough  TsampIntegralVariant=Disabled_SignalSpec  ExternalSaturationOutDataTypeStr=Inherit: Same as second input
      settings: LibrarySourceBlock=simulink/Discrete/Discrete PID Controller
  cfblk4 : Sum  Inputs=|++
  cfblk5 : Gain  Gain=[-72229435.906126]
  cfblk6 : Constant  Value=[804152371.019318]  SampleTime=1
  cfblk7 : Constant  Value=[-638234997.274083]  SampleTime=1
  cfblk2 : Outport
  cfblk13 : Outport  Port=2
  wires:
  cfblk10/1 -> cfblk4/1
  cfblk8/1 -> cfblk3/1
  cfblk5/1 -> cfblk2/1
  cfblk3/1 -> cfblk4/2
  cfblk12/1 -> cfblk5/1
  cfblk4/1 -> cfblk13/1
